simulink model "GestionTermica"  (R2025b)
settings: Solver=VariableStepAuto  StartTime=0.0  StopTime=1100  RelTol=1e-3
libraries: SignalEditorBlockLib x2
settings Model: Creator=usuario  LastModifiedBy=usuario

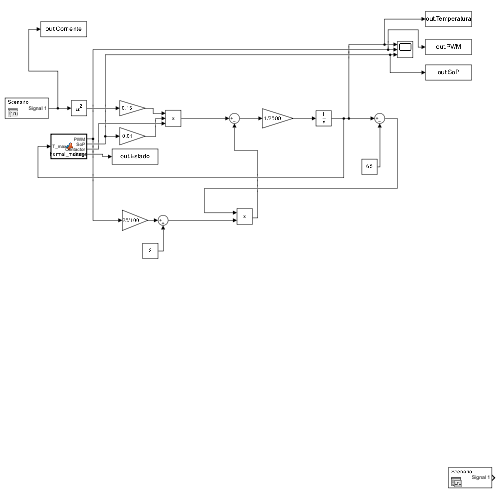
[thumbnail: Simulink's stored preview of the top-level diagram]
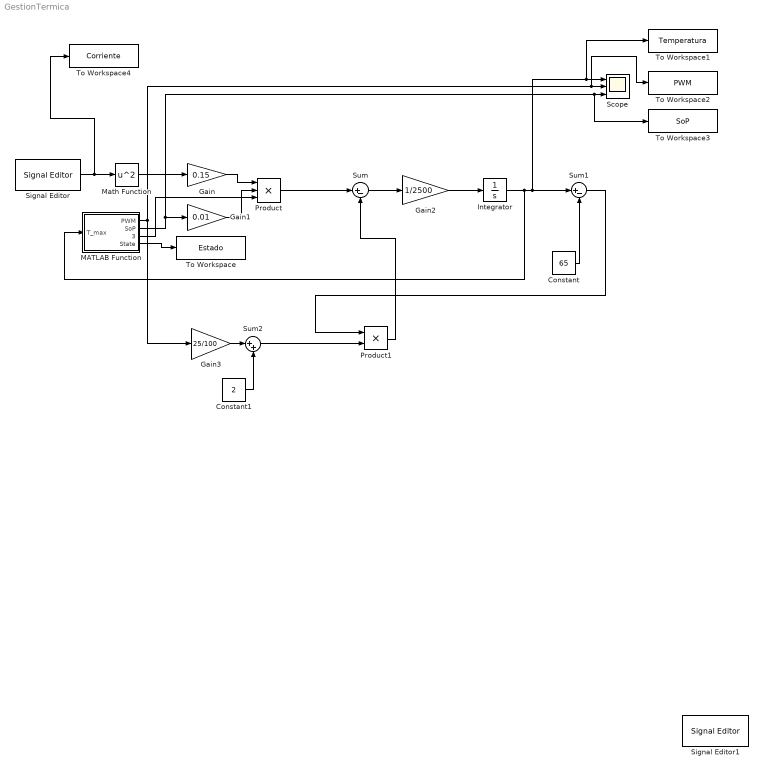
== system GestionTermica ==
  Constant : Constant  Value=65
  Constant1 : Constant  Value=2
  Gain : Gain  Gain=0.15
  Gain1 : Gain  Gain=0.01
  Gain2 : Gain  Gain=1/2500
  Gain3 : Gain  Gain=25/100
  Integrator : Integrator  InitialCondition=20
  MATLAB Function : MATLAB Function  TreatAsAtomicUnit=on  SystemSampleTime=0.1
  Math Function : Math  Operator=square
  Product : Product  Inputs=3
  Product1 : Product
  Scope : Scope  NumInputPorts=3
      settings: ActiveDisplayYMinimum=13.126420990032047  ActiveDisplayYMaximum=81.8622110897116
  Signal Editor : SignalEditorBlockLib/Signal Editor  FileName=untitled.mat  ActiveScenario=Scenario  ActiveSignal=Signal 1  IsBus=off  OutputBusObjectStr=Bus: BusObject  SampleTime=0  ZeroCross=off  OutputAfterFinalValue=Setting to zero  Unit=inherit  PreserveSignalName=on  ApplySigPropsToAllScenarios=on  ApplySigPropsToAllSignals=off  SignalPropertySource=Dialog parameters
  Signal Editor1 : SignalEditorBlockLib/Signal Editor  FileName=untitled.mat  ActiveScenario=Scenario  ActiveSignal=Signal 1  IsBus=off  OutputBusObjectStr=Bus: BusObject  SampleTime=0  ZeroCross=off  OutputAfterFinalValue=Setting to zero  Unit=inherit  PreserveSignalName=on  ApplySigPropsToAllScenarios=on  ApplySigPropsToAllSignals=off  SignalPropertySource=Dialog parameters
  Sum : Sum  Inputs=|+-
  Sum1 : Sum  Inputs=|+-
  Sum2 : Sum  Inputs=|++
  To Workspace : ToWorkspace  VariableName=Estado  SaveFormat=Timeseries  SampleTime=-1
  To Workspace1 : ToWorkspace  VariableName=Temperatura  SaveFormat=Timeseries  SampleTime=-1
  To Workspace2 : ToWorkspace  VariableName=PWM  SaveFormat=Timeseries  SampleTime=-1
  To Workspace3 : ToWorkspace  VariableName=SoP  SaveFormat=Timeseries  SampleTime=-1
  To Workspace4 : ToWorkspace  VariableName=Corriente  SaveFormat=Timeseries  SampleTime=-1
  wires:
  Signal Editor/1 -> To Workspace4/1, Math Function/1
  Math Function/1 -> Gain/1
  Gain/1 -> Product/1
  MATLAB Function/3(Contactor) -> Product/3
  MATLAB Function/2(SoP) -> Gain1/1, To Workspace3/1, Scope/3
  Gain1/1 -> Product/2
  Product/1 -> Sum/1
  Sum/1 -> Gain2/1
  Gain2/1 -> Integrator/1
  Integrator/1 -> To Workspace1/1, Scope/1, Sum1/1, MATLAB Function/1(T_max)
  Constant/1 -> Sum1/2
  Constant1/1 -> Sum2/2
  Gain3/1 -> Sum2/1
  MATLAB Function/1(PWM) -> Gain3/1, To Workspace2/1, Scope/2
  Sum2/1 -> Product1/2
  Sum1/1 -> Product1/1
  Product1/1 -> Sum/2
  MATLAB Function/4(State) -> To Workspace/1

== matlab function GestionTermica/MATLAB Function ==
  data: T_max input; PWM output; SoP output; Contactor output; State output
function [PWM, SoP, Contactor, State] = thermal_manager(T_max)
    % THERMAL_MANAGER: Máquina de estados para gestión térmica del BMS
    
    persistent currentState;
    if isempty(currentState)
        currentState = 1; 
    end

    % =========================================================================
    % --- INICIALIZACIÓN POR DEFECTO (Obligatorio para evitar errores de Coder) ---
    % Damos un valor inicial seguro a las salidas. Si el switch posterior cambia 
    % estos valores, se sobrescribirán perfectamente.
    % =========================================================================
    PWM = 0;
    SoP = 100;
    Contactor = 1;
    % =========================================================================

    % --- DEFINICIÓN DE UMBRALES (Según memoria del TFG) ---
    T_ON       = 35.0; 
    T_OFF      = 32.0; 
    T_SOP_ON   = 50.0; 
    T_CRIT     = 60.0; 
    T_RECOVERY = 50.0; 

    % --- MÁQUINA DE ESTADOS (Transiciones) ---
    switch currentState
        case 1 % Estado 1: Operación Nominal (<35ºC)
            if T_max >= T_ON
                currentState = 2;
            end
            
        case 2 % Estado 2: Advección Proporcional (35ºC - 50ºC)
            if T_max <= T_OFF
                currentState = 1;
            elseif T_max >= T_SOP_ON
                currentState = 3;
            end
            
        case 3 % Estado 3: Limitación de Potencia (50ºC - 60ºC)
            if T_max < T_SOP_ON
                currentState = 2;
            elseif T_max >= T_CRIT
                currentState = 4;
            end
            
        case 4 % Estado 4: Parada de Emergencia (>=60ºC)
            if T_max <= T_RECOVERY
                currentState = 3; 
            end
    end

    % --- LÓGICA DE CONTROL (Acciones según el estado) ---
    switch currentState
        case 1
            PWM = 0;
            SoP = 100;
            Contactor = 1;
            
        case 2
            PWM = 30 + 4.67 * (T_max - T_ON);
            if PWM > 100
                PWM = 100; 
            elseif PWM < 30
                PWM = 30;
            end
            SoP = 100;
            Contactor = 1;
            
        case 3
            PWM = 100; 
            SoP = 100 - ((T_max - T_SOP_ON) * 10);
            if SoP < 0
                SoP = 0; 
            end
            Contactor = 1;
            
        case 4
            PWM = 100;  
            SoP = 0;    
            Contactor = 0; 
    end

    % Salida de diagnóstico
    State = currentState;
end
